simulink model "LUT_liver_pancreas_30"  (R2023b)
settings: Solver=FixedStepAuto  StartTime=0  StopTime=10.1  FixedStep=Timegap  RelTol=1e-3
model workspace (MAT data in the model file):
  T1_input = 1.34
(part 2 of 3)

== system LUT_liver_pancreas_30/If Action Subsystem6/If Action Subsystem1/If Action Subsystem6/If Action Subsystem3 ==
  In1 : Inport
  Action Port : ActionPort  ActionPortLabel=elseif( u1 >= 1.025)
  LUT 1.03RR : Lookup_n-D  NumberOfTableDimensions=1  BreakpointsForDimension1=[465.6797;513.9306;612.0294;710.55;809.0188;907.4097;1005.737;1104.014;1202.255;1300.466;1398.654;1496.822;1594.973;1693.109;1791.227;1889.324;1987.387]  Table=[400;500;600;700;800;900;1000;1100;1200;1300;1400;1500;1600;1700;1800;1900;2000]  InternalRulePriority=Speed  RndMeth=Simplest
  Out1 : Outport
  wires:
  In1/1 -> LUT 1.03RR/1
  LUT 1.03RR/1 -> Out1/1

== system LUT_liver_pancreas_30/If Action Subsystem6/If Action Subsystem1/If Action Subsystem6/If Action Subsystem4 ==
  In1 : Inport
  Action Port : ActionPort  ActionPortLabel=elseif( u1 >= 1.035)
  LUT 1.04RR : Lookup_n-D  NumberOfTableDimensions=1  BreakpointsForDimension1=[465.4805;513.7116;611.7076;710.1164;808.4681;906.7384;1004.942;1103.096;1201.21;1299.295;1397.356;1495.397;1593.421;1691.429;1789.421;1887.393;1985.334]  Table=[400;500;600;700;800;900;1000;1100;1200;1300;1400;1500;1600;1700;1800;1900;2000]  InternalRulePriority=Speed  RndMeth=Simplest
  Out1 : Outport
  wires:
  In1/1 -> LUT 1.04RR/1
  LUT 1.04RR/1 -> Out1/1

== system LUT_liver_pancreas_30/If Action Subsystem6/If Action Subsystem1/If Action Subsystem6/If Action Subsystem5 ==
  In1 : Inport
  Action Port : ActionPort  ActionPortLabel=elseif( u1 >= 1.055)
  LUT 1.06RR : Lookup_n-D  NumberOfTableDimensions=1  BreakpointsForDimension1=[465.091;513.2858;611.0845;709.278;807.4037;905.441;1003.407;1101.319;1199.191;1297.031;1394.845;1492.639;1590.416;1688.177;1785.923;1883.65;1981.353]  Table=[400;500;600;700;800;900;1000;1100;1200;1300;1400;1500;1600;1700;1800;1900;2000]  InternalRulePriority=Speed  RndMeth=Simplest
  Out1 : Outport
  wires:
  In1/1 -> LUT 1.06RR/1
  LUT 1.06RR/1 -> Out1/1

== system LUT_liver_pancreas_30/If Action Subsystem6/If Action Subsystem1/If Action Subsystem6/If Action Subsystem6 ==
  In1 : Inport
  Action Port : ActionPort  ActionPortLabel=elseif( u1 >= 1.045)
  LUT 1.05RR : Lookup_n-D  NumberOfTableDimensions=1  BreakpointsForDimension1=[465.2843;513.4967;611.3927;709.6925;807.9298;906.0823;1004.166;1102.198;1200.189;1298.15;1396.087;1494.003;1591.902;1689.785;1787.653;1885.502;1983.323]  Table=[400;500;600;700;800;900;1000;1100;1200;1300;1400;1500;1600;1700;1800;1900;2000]  InternalRulePriority=Speed  RndMeth=Simplest
  Out1 : Outport
  wires:
  In1/1 -> LUT 1.05RR/1
  LUT 1.05RR/1 -> Out1/1

== system LUT_liver_pancreas_30/If Action Subsystem6/If Action Subsystem1/If Action Subsystem6/If Action Subsystem7 ==
  In1 : Inport
  Action Port : ActionPort  ActionPortLabel=elseif( u1 >= 1.065)
  LUT 1.07RR : Lookup_n-D  NumberOfTableDimensions=1  BreakpointsForDimension1=[464.9007;513.0789;610.783;708.8729;806.8895;904.8142;1002.665;1100.461;1198.214;1295.935;1393.631;1491.305;1588.962;1686.603;1784.229;1881.838;1979.424]  Table=[400;500;600;700;800;900;1000;1100;1200;1300;1400;1500;1600;1700;1800;1900;2000]  InternalRulePriority=Speed  RndMeth=Simplest
  Out1 : Outport
  wires:
  In1/1 -> LUT 1.07RR/1
  LUT 1.07RR/1 -> Out1/1

== system LUT_liver_pancreas_30/If Action Subsystem6/If Action Subsystem1/If Action Subsystem6/If Action Subsystem8 ==
  In1 : Inport
  Action Port : ActionPort  ActionPortLabel=elseif(u1 >= 1.075)
  LUT 1.08RR : Lookup_n-D  NumberOfTableDimensions=1  BreakpointsForDimension1=[464.7133;512.876;610.4881;708.4768;806.3869;904.2015;1001.94;1099.622;1197.26;1294.864;1392.443;1490;1587.539;1685.063;1782.571;1880.063;1977.535]  Table=[400;500;600;700;800;900;1000;1100;1200;1300;1400;1500;1600;1700;1800;1900;2000]  InternalRulePriority=Speed  RndMeth=Simplest
  Out1 : Outport
  wires:
  In1/1 -> LUT 1.08RR/1
  LUT 1.08RR/1 -> Out1/1

== system LUT_liver_pancreas_30/If Action Subsystem6/If Action Subsystem1/If Action Subsystem6/If Action Subsystem9 ==
  In1 : Inport
  Action Port : ActionPort  ActionPortLabel=if(u1 >= 1.085)
  LUT 1.09RR : Lookup_n-D  NumberOfTableDimensions=1  BreakpointsForDimension1=[412.0667;553.6807;651.0883;748.3345;845.4429;942.4605;1039.419;1136.338;1233.23;1330.102;1426.961;1523.81;1620.651;1717.486;1814.317;1911.142;2007.964]  Table=[464.5288;512.6769;610.1995;708.0897;805.8957;903.6027;1001.231;1098.801;1196.326;1293.817;1391.281;1488.723;1586.147;1683.555;1780.949;1878.326;1975.684]  InternalRulePriority=Speed  RndMeth=Simplest
  Out1 : Outport
  wires:
  In1/1 -> LUT 1.09RR/1
  LUT 1.09RR/1 -> Out1/1

== system LUT_liver_pancreas_30/If Action Subsystem6/If Action Subsystem1/If Action Subsystem7/If Action Subsystem1 ==
  In1 : Inport
  Action Port : ActionPort  ActionPortLabel=elseif( u1 >= 1.215)
  LUT 1.22RR : Lookup_n-D  NumberOfTableDimensions=1  BreakpointsForDimension1=[462.3821;510.4145;606.9721;703.7795;800.4299;896.9327;993.3239;1089.632;1185.879;1282.079;1378.243;1474.378;1570.491;1666.584;1762.661;1858.723;1954.773]  Table=[400;500;600;700;800;900;1000;1100;1200;1300;1400;1500;1600;1700;1800;1900;2000]  InternalRulePriority=Speed  RndMeth=Simplest
  Out1 : Outport
  wires:
  In1/1 -> LUT 1.22RR/1
  LUT 1.22RR/1 -> Out1/1

== system LUT_liver_pancreas_30/If Action Subsystem6/If Action Subsystem1/If Action Subsystem7/If Action Subsystem10 ==
  In1 : Inport
  Action Port : ActionPort  ActionPortLabel=elseif( u1 >= 1.205)
  LUT 1.21RR : Lookup_n-D  NumberOfTableDimensions=1  BreakpointsForDimension1=[462.5316;510.5687;607.1891;704.0681;800.7958;897.3798;993.8548;1090.249;1186.583;1282.871;1379.124;1475.349;1571.551;1667.734;1763.902;1860.055;1956.195]  Table=[400;500;600;700;800;900;1000;1100;1200;1300;1400;1500;1600;1700;1800;1900;2000]  InternalRulePriority=Speed  RndMeth=Simplest
  Out1 : Outport
  wires:
  In1/1 -> LUT 1.21RR/1
  LUT 1.21RR/1 -> Out1/1

== system LUT_liver_pancreas_30/If Action Subsystem6/If Action Subsystem1/If Action Subsystem7/If Action Subsystem2 ==
  In1 : Inport
  Action Port : ActionPort  ActionPortLabel=else
  LUT 1.20RR : Lookup_n-D  NumberOfTableDimensions=1  BreakpointsForDimension1=[462.6836;510.7261;607.4108;704.3632;801.17;897.8369;994.3974;1090.879;1187.302;1283.68;1380.023;1476.339;1572.633;1668.908;1765.168;1861.413;1957.645]  Table=[400;500;600;700;800;900;1000;1100;1200;1300;1400;1500;1600;1700;1800;1900;2000]  InternalRulePriority=Speed  RndMeth=Simplest
  Out1 : Outport
  wires:
  In1/1 -> LUT 1.20RR/1
  LUT 1.20RR/1 -> Out1/1

== system LUT_liver_pancreas_30/If Action Subsystem6/If Action Subsystem1/If Action Subsystem7/If Action Subsystem3 ==
  In1 : Inport
  Action Port : ActionPort  ActionPortLabel=elseif( u1 >= 1.225)
  LUT 1.23RR : Lookup_n-D  NumberOfTableDimensions=1  BreakpointsForDimension1=[462.235;510.2632;606.7599;703.4974;800.072;896.4954;992.8044;1089.029;1185.19;1281.304;1377.38;1473.428;1569.452;1665.456;1761.444;1857.418;1953.378]  Table=[400;500;600;700;800;900;1000;1100;1200;1300;1400;1500;1600;1700;1800;1900;2000]  InternalRulePriority=Speed  RndMeth=Simplest
  Out1 : Outport
  wires:
  In1/1 -> LUT 1.23RR/1
  LUT 1.23RR/1 -> Out1/1

== system LUT_liver_pancreas_30/If Action Subsystem6/If Action Subsystem1/If Action Subsystem7/If Action Subsystem4 ==
  In1 : Inport
  Action Port : ActionPort  ActionPortLabel=elseif( u1 >= 1.235)
  LUT 1.24RR : Lookup_n-D  NumberOfTableDimensions=1  BreakpointsForDimension1=[462.0903;510.1148;606.5523;703.2214;799.7221;896.0676;992.296;1088.438;1184.516;1280.544;1376.535;1472.496;1568.433;1664.351;1760.251;1856.137;1952.01]  Table=[400;500;600;700;800;900;1000;1100;1200;1300;1400;1500;1600;1700;1800;1900;2000]  InternalRulePriority=Speed  RndMeth=Simplest
  Out1 : Outport
  wires:
  In1/1 -> LUT 1.24RR/1
  LUT 1.24RR/1 -> Out1/1

== system LUT_liver_pancreas_30/If Action Subsystem6/If Action Subsystem1/If Action Subsystem7/If Action Subsystem5 ==
  In1 : Inport
  Action Port : ActionPort  ActionPortLabel=elseif( u1 >= 1.255)
  LUT 1.26RR : Lookup_n-D  NumberOfTableDimensions=1  BreakpointsForDimension1=[461.8078;509.8267;606.1502;702.6876;799.045;895.2396;991.3117;1087.293;1183.208;1279.071;1374.896;1470.689;1566.457;1662.204;1757.935;1853.651;1949.353]  Table=[400;500;600;700;800;900;1000;1100;1200;1300;1400;1500;1600;1700;1800;1900;2000]  InternalRulePriority=Speed  RndMeth=Simplest
  Out1 : Outport
  wires:
  In1/1 -> LUT 1.26RR/1
  LUT 1.26RR/1 -> Out1/1

== system LUT_liver_pancreas_30/If Action Subsystem6/If Action Subsystem1/If Action Subsystem7/If Action Subsystem6 ==
  In1 : Inport
  Action Port : ActionPort  ActionPortLabel=elseif( u1 >= 1.245)
  LUT 1.25RR : Lookup_n-D  NumberOfTableDimensions=1  BreakpointsForDimension1=[461.9479;509.9694;606.349;702.9515;799.3798;895.6491;991.7985;1087.86;1183.855;1279.8;1375.707;1471.583;1567.435;1663.267;1759.082;1854.882;1950.669]  Table=[400;500;600;700;800;900;1000;1100;1200;1300;1400;1500;1600;1700;1800;1900;2000]  InternalRulePriority=Speed  RndMeth=Simplest
  Out1 : Outport
  wires:
  In1/1 -> LUT 1.25RR/1
  LUT 1.25RR/1 -> Out1/1

== system LUT_liver_pancreas_30/If Action Subsystem6/If Action Subsystem1/If Action Subsystem7/If Action Subsystem7 ==
  In1 : Inport
  Action Port : ActionPort  ActionPortLabel=elseif( u1 >= 1.265)
  LUT 1.27RR : Lookup_n-D  NumberOfTableDimensions=1  BreakpointsForDimension1=[461.6699;509.6867;605.9556;702.4294;798.7176;894.839;990.8352;1086.739;1182.574;1278.357;1374.1;1469.812;1565.498;1661.163;1756.81;1852.443;1948.062]  Table=[400;500;600;700;800;900;1000;1100;1200;1300;1400;1500;1600;1700;1800;1900;2000]  InternalRulePriority=Speed  RndMeth=Simplest
  Out1 : Outport
  wires:
  In1/1 -> LUT 1.27RR/1
  LUT 1.27RR/1 -> Out1/1

== system LUT_liver_pancreas_30/If Action Subsystem6/If Action Subsystem1/If Action Subsystem7/If Action Subsystem8 ==
  In1 : Inport
  Action Port : ActionPort  ActionPortLabel=elseif(u1 >= 1.275)
  LUT 1.28RR : Lookup_n-D  NumberOfTableDimensions=1  BreakpointsForDimension1=[461.5343;509.5495;605.7652;702.1769;798.3973;894.447;990.3687;1086.196;1181.954;1277.658;1373.321;1468.952;1564.557;1660.141;1755.707;1851.258;1946.796]  Table=[400;500;600;700;800;900;1000;1100;1200;1300;1400;1500;1600;1700;1800;1900;2000]  InternalRulePriority=Speed  RndMeth=Simplest
  Out1 : Outport
  wires:
  In1/1 -> LUT 1.28RR/1
  LUT 1.28RR/1 -> Out1/1

== system LUT_liver_pancreas_30/If Action Subsystem6/If Action Subsystem1/If Action Subsystem7/If Action Subsystem9 ==
  In1 : Inport
  Action Port : ActionPort  ActionPortLabel=if(u1 >= 1.285)
  LUT 1.29RR : Lookup_n-D  NumberOfTableDimensions=1  BreakpointsForDimension1=[461.4008;509.4148;605.5788;701.9299;798.084;894.0634;989.9122;1085.665;1181.346;1276.973;1372.558;1468.11;1563.635;1659.139;1754.625;1850.096;1945.553]  Table=[400;500;600;700;800;900;1000;1100;1200;1300;1400;1500;1600;1700;1800;1900;2000]  InternalRulePriority=Speed  RndMeth=Simplest
  Out1 : Outport
  wires:
  In1/1 -> LUT 1.29RR/1
  LUT 1.29RR/1 -> Out1/1

== system LUT_liver_pancreas_30/If Action Subsystem6/If Action Subsystem1/If Action Subsystem8/If Action Subsystem1 ==
  In1 : Inport
  Action Port : ActionPort  ActionPortLabel=elseif( u1 >= 1.315)
  LUT 1.32RR : Lookup_n-D  NumberOfTableDimensions=1  BreakpointsForDimension1=[461.0128;509.0261;605.043;701.2207;797.1841;892.9612;988.5993;1084.135;1179.595;1274.998;1370.356;1465.679;1560.975;1656.247;1751.501;1846.739;1941.963]  Table=[400;500;600;700;800;900;1000;1100;1200;1300;1400;1500;1600;1700;1800;1900;2000]  InternalRulePriority=Speed  RndMeth=Simplest
  Out1 : Outport
  wires:
  In1/1 -> LUT 1.32RR/1
  LUT 1.32RR/1 -> Out1/1

== system LUT_liver_pancreas_30/If Action Subsystem6/If Action Subsystem1/If Action Subsystem8/If Action Subsystem10 ==
  In1 : Inport
  Action Port : ActionPort  ActionPortLabel=elseif( u1 >= 1.305)
  LUT 1.31RR : Lookup_n-D  NumberOfTableDimensions=1  BreakpointsForDimension1=[461.1401;509.1532;605.2178;701.452;797.4775;893.3207;989.0277;1084.635;1180.167;1275.643;1371.075;1466.474;1561.844;1657.193;1752.523;1847.837;1943.137]  Table=[400;500;600;700;800;900;1000;1100;1200;1300;1400;1500;1600;1700;1800;1900;2000]  InternalRulePriority=Speed  RndMeth=Simplest
  Out1 : Outport
  wires:
  In1/1 -> LUT 1.31RR/1
  LUT 1.31RR/1 -> Out1/1

== system LUT_liver_pancreas_30/If Action Subsystem6/If Action Subsystem1/If Action Subsystem8/If Action Subsystem2 ==
  In1 : Inport
  Action Port : ActionPort  ActionPortLabel=else
  LUT 1.30RR : Lookup_n-D  NumberOfTableDimensions=1  BreakpointsForDimension1=[461.2694;509.2828;605.3963;701.6863;797.7774;893.688;989.4652;1085.144;1180.75;1276.301;1371.809;1467.283;1562.731;1658.157;1753.564;1848.956;1944.334]  Table=[400;500;600;700;800;900;1000;1100;1200;1300;1400;1500;1600;1700;1800;1900;2000]  InternalRulePriority=Speed  RndMeth=Simplest
  Out1 : Outport
  wires:
  In1/1 -> LUT 1.30RR/1
  LUT 1.30RR/1 -> Out1/1

== system LUT_liver_pancreas_30/If Action Subsystem6/If Action Subsystem1/If Action Subsystem8/If Action Subsystem3 ==
  In1 : Inport
  Action Port : ActionPort  ActionPortLabel=elseif( u1 >= 1.325)
  LUT 1.33RR : Lookup_n-D  NumberOfTableDimensions=1  BreakpointsForDimension1=[460.8876;508.9014;604.8719;700.9945;796.897;892.6093;988.1798;1083.646;1179.035;1274.366;1369.651;1464.9;1560.122;1655.32;1750.499;1845.662;1940.81]  Table=[400;500;600;700;800;900;1000;1100;1200;1300;1400;1500;1600;1700;1800;1900;2000]  InternalRulePriority=Speed  RndMeth=Simplest
  Out1 : Outport
  wires:
  In1/1 -> LUT 1.33RR/1
  LUT 1.33RR/1 -> Out1/1

== system LUT_liver_pancreas_30/If Action Subsystem6/If Action Subsystem1/If Action Subsystem8/If Action Subsystem4 ==
  In1 : Inport
  Action Port : ActionPort  ActionPortLabel=elseif( u1 >= 1.335)
  LUT 1.34RR : Lookup_n-D  NumberOfTableDimensions=1  BreakpointsForDimension1=[460.7643;508.779;604.7044;700.7732;796.6161;892.2649;987.7691;1083.167;1178.486;1273.746;1368.959;1464.137;1559.285;1654.41;1749.515;1844.604;1939.678]  Table=[400;500;600;700;800;900;1000;1100;1200;1300;1400;1500;1600;1700;1800;1900;2000]  InternalRulePriority=Speed  RndMeth=Simplest
  Out1 : Outport
  wires:
  In1/1 -> LUT 1.34RR/1
  LUT 1.34RR/1 -> Out1/1

== system LUT_liver_pancreas_30/If Action Subsystem6/If Action Subsystem1/If Action Subsystem8/If Action Subsystem5 ==
  In1 : Inport
  Action Port : ActionPort  ActionPortLabel=elseif( u1 >= 1.355)
  LUT 1.36RR : Lookup_n-D  NumberOfTableDimensions=1  BreakpointsForDimension1=[460.5234;508.5411;604.3798;700.3447;796.0723;891.5977;986.9731;1082.238;1177.422;1272.543;1367.616;1462.652;1557.658;1652.64;1747.602;1842.547;1937.477]  Table=[400;500;600;700;800;900;1000;1100;1200;1300;1400;1500;1600;1700;1800;1900;2000]  InternalRulePriority=Speed  RndMeth=Simplest
  Out1 : Outport
  wires:
  In1/1 -> LUT 1.36RR/1
  LUT 1.36RR/1 -> Out1/1

== system LUT_liver_pancreas_30/If Action Subsystem6/If Action Subsystem1/If Action Subsystem8/If Action Subsystem6 ==
  In1 : Inport
  Action Port : ActionPort  ActionPortLabel=elseif( u1 >= 1.345)
  LUT 1.35RR : Lookup_n-D  NumberOfTableDimensions=1  BreakpointsForDimension1=[460.6429;508.6589;604.5404;700.5566;796.3413;891.9277;987.3669;1082.698;1177.949;1273.138;1368.281;1463.387;1558.464;1653.517;1748.55;1843.566;1938.567]  Table=[400;500;600;700;800;900;1000;1100;1200;1300;1400;1500;1600;1700;1800;1900;2000]  InternalRulePriority=Speed  RndMeth=Simplest
  Out1 : Outport
  wires:
  In1/1 -> LUT 1.35RR/1
  LUT 1.35RR/1 -> Out1/1

== system LUT_liver_pancreas_30/If Action Subsystem6/If Action Subsystem1/If Action Subsystem8/If Action Subsystem7 ==
  In1 : Inport
  Action Port : ActionPort  ActionPortLabel=elseif( u1 >= 1.365)
  LUT 1.37RR : Lookup_n-D  NumberOfTableDimensions=1  BreakpointsForDimension1=[460.4057;508.4254;604.2226;700.1373;795.809;891.2746;986.5873;1081.788;1176.905;1271.959;1366.964;1461.932;1556.868;1651.78;1746.672;1841.546;1936.405]  Table=[400;500;600;700;800;900;1000;1100;1200;1300;1400;1500;1600;1700;1800;1900;2000]  InternalRulePriority=Speed  RndMeth=Simplest
  Out1 : Outport
  wires:
  In1/1 -> LUT 1.37RR/1
  LUT 1.37RR/1 -> Out1/1

== system LUT_liver_pancreas_30/If Action Subsystem6/If Action Subsystem1/If Action Subsystem8/If Action Subsystem8 ==
  In1 : Inport
  Action Port : ActionPort  ActionPortLabel=elseif(u1 >= 1.375)
  LUT 1.38RR : Lookup_n-D  NumberOfTableDimensions=1  BreakpointsForDimension1=[460.2899;508.3119;604.0687;699.9344;795.5514;890.9583;986.2096;1081.347;1176.399;1271.386;1366.325;1461.224;1556.093;1650.936;1745.758;1840.564;1935.354]  Table=[400;500;600;700;800;900;1000;1100;1200;1300;1400;1500;1600;1700;1800;1900;2000]  InternalRulePriority=Speed  RndMeth=Simplest
  Out1 : Outport
  wires:
  In1/1 -> LUT 1.38RR/1
  LUT 1.38RR/1 -> Out1/1

== system LUT_liver_pancreas_30/If Action Subsystem6/If Action Subsystem1/If Action Subsystem8/If Action Subsystem9 ==
  In1 : Inport
  Action Port : ActionPort  ActionPortLabel=if(u1 >= 1.385)
  LUT 1.39RR : Lookup_n-D  NumberOfTableDimensions=1  BreakpointsForDimension1=[460.1758;508.2005;603.9179;699.7359;795.2993;890.6487;985.8396;1080.914;1175.902;1270.825;1365.698;1460.53;1555.332;1650.107;1744.862;1839.599;1934.321]  Table=[400;500;600;700;800;900;1000;1100;1200;1300;1400;1500;1600;1700;1800;1900;2000]  InternalRulePriority=Speed  RndMeth=Simplest
  Out1 : Outport
  wires:
  In1/1 -> LUT 1.39RR/1
  LUT 1.39RR/1 -> Out1/1

== system LUT_liver_pancreas_30/If Action Subsystem6/If Action Subsystem1/If Action Subsystem9/If Action Subsystem1 ==
  In1 : Inport
  Action Port : ActionPort  ActionPortLabel=elseif( u1 >= 1.415)
  LUT 1.42RR : Lookup_n-D  NumberOfTableDimensions=1  BreakpointsForDimension1=[459.8439;507.8784;603.4841;699.1652;794.5746;889.758;984.7744;1079.668;1174.471;1269.205;1363.886;1458.526;1553.132;1647.711;1742.269;1836.807;1931.33]  Table=[400;500;600;700;800;900;1000;1100;1200;1300;1400;1500;1600;1700;1800;1900;2000]  InternalRulePriority=Speed  RndMeth=Simplest
  Out1 : Outport
  wires:
  In1/1 -> LUT 1.42RR/1
  LUT 1.42RR/1 -> Out1/1

== system LUT_liver_pancreas_30/If Action Subsystem6/If Action Subsystem1/If Action Subsystem9/If Action Subsystem10 ==
  In1 : Inport
  Action Port : ActionPort  ActionPortLabel=elseif( u1 >= 1.405)
  LUT 1.41RR : Lookup_n-D  NumberOfTableDimensions=1  BreakpointsForDimension1=[459.9529;507.9838;603.6257;699.3513;794.811;890.0486;985.1221;1080.075;1174.939;1269.735;1364.479;1459.181;1553.852;1648.495;1743.117;1837.721;1932.309]  Table=[400;500;600;700;800;900;1000;1100;1200;1300;1400;1500;1600;1700;1800;1900;2000]  InternalRulePriority=Speed  RndMeth=Simplest
  Out1 : Outport
  wires:
  In1/1 -> LUT 1.41RR/1
  LUT 1.41RR/1 -> Out1/1

== system LUT_liver_pancreas_30/If Action Subsystem6/If Action Subsystem1/If Action Subsystem9/If Action Subsystem2 ==
  In1 : Inport
  Action Port : ActionPort  ActionPortLabel=else
  LUT 1.40RR : Lookup_n-D  NumberOfTableDimensions=1  BreakpointsForDimension1=[460.0635;508.0912;603.7703;699.5415;795.0525;890.3455;985.4771;1080.49;1175.416;1270.275;1365.082;1459.85;1554.585;1649.294;1743.982;1838.651;1933.306]  Table=[400;500;600;700;800;900;1000;1100;1200;1300;1400;1500;1600;1700;1800;1900;2000]  InternalRulePriority=Speed  RndMeth=Simplest
  Out1 : Outport
  wires:
  In1/1 -> LUT 1.40RR/1
  LUT 1.40RR/1 -> Out1/1

== system LUT_liver_pancreas_30/If Action Subsystem6/If Action Subsystem1/If Action Subsystem9/If Action Subsystem3 ==
  In1 : Inport
  Action Port : ActionPort  ActionPortLabel=elseif( u1 >= 1.425)
  LUT 1.43RR : Lookup_n-D  NumberOfTableDimensions=1  BreakpointsForDimension1=[459.7366;507.7749;603.3454;698.9829;794.3431;889.4733;984.4337;1079.27;1174.013;1268.686;1363.305;1457.882;1552.426;1646.942;1741.435;1835.91;1930.368]  Table=[400;500;600;700;800;900;1000;1100;1200;1300;1400;1500;1600;1700;1800;1900;2000]  InternalRulePriority=Speed  RndMeth=Simplest
  Out1 : Outport
  wires:
  In1/1 -> LUT 1.43RR/1
  LUT 1.43RR/1 -> Out1/1

== system LUT_liver_pancreas_30/If Action Subsystem6/If Action Subsystem1/If Action Subsystem9/If Action Subsystem4 ==
  In1 : Inport
  Action Port : ActionPort  ActionPortLabel=elseif( u1 >= 1.435)
  LUT 1.44RR : Lookup_n-D  NumberOfTableDimensions=1  BreakpointsForDimension1=[459.6309;507.6733;603.2096;698.8046;794.1166;889.1946;984.1;1078.879;1173.563;1268.177;1362.735;1457.251;1551.732;1646.186;1740.616;1835.028;1929.423]  Table=[400;500;600;700;800;900;1000;1100;1200;1300;1400;1500;1600;1700;1800;1900;2000]  InternalRulePriority=Speed  RndMeth=Simplest
  Out1 : Outport
  wires:
  In1/1 -> LUT 1.44RR/1
  LUT 1.44RR/1 -> Out1/1

== system LUT_liver_pancreas_30/If Action Subsystem6/If Action Subsystem1/If Action Subsystem9/If Action Subsystem5 ==
  In1 : Inport
  Action Port : ActionPort  ActionPortLabel=elseif( u1 >= 1.455)
  LUT 1.46RR : Lookup_n-D  NumberOfTableDimensions=1  BreakpointsForDimension1=[459.4241;507.4755;602.9462;698.4591;793.6778;888.6544;983.4526;1078.12;1172.69;1267.187;1361.627;1456.023;1550.383;1644.714;1739.022;1833.311;1927.583]  Table=[400;500;600;700;800;900;1000;1100;1200;1300;1400;1500;1600;1700;1800;1900;2000]  InternalRulePriority=Speed  RndMeth=Simplest
  Out1 : Outport
  wires:
  In1/1 -> LUT 1.46RR/1
  LUT 1.46RR/1 -> Out1/1

== system LUT_liver_pancreas_30/If Action Subsystem6/If Action Subsystem1/If Action Subsystem9/If Action Subsystem6 ==
  In1 : Inport
  Action Port : ActionPort  ActionPortLabel=elseif( u1 >= 1.445)
  LUT 1.45RR : Lookup_n-D  NumberOfTableDimensions=1  BreakpointsForDimension1=[459.5267;507.5735;603.0765;698.63;793.8948;888.9217;983.773;1078.496;1173.123;1267.677;1362.176;1456.631;1551.051;1645.443;1739.812;1834.162;1928.495]  Table=[400;500;600;700;800;900;1000;1100;1200;1300;1400;1500;1600;1700;1800;1900;2000]  InternalRulePriority=Speed  RndMeth=Simplest
  Out1 : Outport
  wires:
  In1/1 -> LUT 1.45RR/1
  LUT 1.45RR/1 -> Out1/1

== system LUT_liver_pancreas_30/If Action Subsystem6/If Action Subsystem1/If Action Subsystem9/If Action Subsystem7 ==
  In1 : Inport
  Action Port : ActionPort  ActionPortLabel=elseif( u1 >= 1.465)
  LUT 1.47RR : Lookup_n-D  NumberOfTableDimensions=1  BreakpointsForDimension1=[459.323;507.3793;602.8185;698.2919;793.4652;888.3926;983.1387;1077.752;1172.266;1266.706;1361.088;1455.425;1549.727;1643.999;1738.247;1832.475;1926.686]  Table=[400;500;600;700;800;900;1000;1100;1200;1300;1400;1500;1600;1700;1800;1900;2000]  InternalRulePriority=Speed  RndMeth=Simplest
  Out1 : Outport
  wires:
  In1/1 -> LUT 1.47RR/1
  LUT 1.47RR/1 -> Out1/1

== system LUT_liver_pancreas_30/If Action Subsystem6/If Action Subsystem1/If Action Subsystem9/If Action Subsystem8 ==
  In1 : Inport
  Action Port : ActionPort  ActionPortLabel=elseif(u1 >= 1.475)
  LUT 1.48RR : Lookup_n-D  NumberOfTableDimensions=1  BreakpointsForDimension1=[459.2234;507.2847;602.6934;698.1281;793.2572;888.1363;982.8312;1077.391;1171.851;1266.235;1360.56;1454.839;1549.082;1643.295;1737.484;1831.653;1925.805]  Table=[400;500;600;700;800;900;1000;1100;1200;1300;1400;1500;1600;1700;1800;1900;2000]  InternalRulePriority=Speed  RndMeth=Simplest
  Out1 : Outport
  wires:
  In1/1 -> LUT 1.48RR/1
  LUT 1.48RR/1 -> Out1/1

== system LUT_liver_pancreas_30/If Action Subsystem6/If Action Subsystem1/If Action Subsystem9/If Action Subsystem9 ==
  In1 : Inport
  Action Port : ActionPort  ActionPortLabel=if(u1 >= 1.485)
  LUT 1.49RR : Lookup_n-D  NumberOfTableDimensions=1  BreakpointsForDimension1=[459.1252;507.1919;602.5709;697.9678;793.0535;887.8852;982.5299;1077.037;1171.443;1265.772;1360.041;1454.264;1548.449;1642.605;1736.735;1830.846;1924.939]  Table=[400;500;600;700;800;900;1000;1100;1200;1300;1400;1500;1600;1700;1800;1900;2000]  InternalRulePriority=Speed  RndMeth=Simplest
  Out1 : Outport
  wires:
  In1/1 -> LUT 1.49RR/1
  LUT 1.49RR/1 -> Out1/1

== system LUT_liver_pancreas_30/If Action Subsystem6/If Action Subsystem2/If Action Subsystem5/If Action Subsystem1 ==
  In1 : Inport
  Action Port : ActionPort  ActionPortLabel=elseif( u1 >= 1.615)
  LUT 1.62RR : Lookup_n-D  NumberOfTableDimensions=1  BreakpointsForDimension1=[457.9682;506.1215;601.1841;696.1646;790.7619;885.0533;979.1199;1073.022;1166.801;1260.486;1354.101;1447.659;1541.172;1634.649;1728.096;1821.519;1914.921]  Table=[400;500;600;700;800;900;1000;1100;1200;1300;1400;1500;1600;1700;1800;1900;2000]  InternalRulePriority=Speed  RndMeth=Simplest
  Out1 : Outport
  wires:
  In1/1 -> LUT 1.62RR/1
  LUT 1.62RR/1 -> Out1/1

== system LUT_liver_pancreas_30/If Action Subsystem6/If Action Subsystem2/If Action Subsystem5/If Action Subsystem10 ==
  In1 : Inport
  Action Port : ActionPort  ActionPortLabel=elseif( u1>= 1.605)
  LUT 1.61RR : Lookup_n-D  NumberOfTableDimensions=1  BreakpointsForDimension1=[458.05;506.1956;601.2784;696.2865;790.9167;885.2451;979.3517;1073.295;1167.118;1260.849;1354.509;1448.114;1541.674;1635.199;1728.694;1822.165;1915.616]  Table=[400;500;600;700;800;900;1000;1100;1200;1300;1400;1500;1600;1700;1800;1900;2000]  InternalRulePriority=Speed  RndMeth=Simplest
  Out1 : Outport
  wires:
  In1/1 -> LUT 1.61RR/1
  LUT 1.61RR/1 -> Out1/1

== system LUT_liver_pancreas_30/If Action Subsystem6/If Action Subsystem2/If Action Subsystem5/If Action Subsystem2 ==
  In1 : Inport
  Action Port : ActionPort  ActionPortLabel=else
  LUT 1.60RR : Lookup_n-D  NumberOfTableDimensions=1  BreakpointsForDimension1=[458.1329;506.271;601.3746;696.4109;791.0749;885.441;979.5882;1073.575;1167.442;1261.218;1354.925;1448.577;1542.185;1635.759;1729.303;1822.823;1916.324]  Table=[400;500;600;700;800;900;1000;1100;1200;1300;1400;1500;1600;1700;1800;1900;2000]  InternalRulePriority=Speed  RndMeth=Simplest
  Out1 : Outport
  wires:
  In1/1 -> LUT 1.60RR/1
  LUT 1.60RR/1 -> Out1/1

== system LUT_liver_pancreas_30/If Action Subsystem6/If Action Subsystem2/If Action Subsystem5/If Action Subsystem3 ==
  In1 : Inport
  Action Port : ActionPort  ActionPortLabel=elseif( u1 >= 1.625)
  LUT 1.63RR : Lookup_n-D  NumberOfTableDimensions=1  BreakpointsForDimension1=[457.8875;506.0486;601.0917;696.0453;790.6102;884.8653;978.8927;1072.753;1166.489;1260.131;1353.7;1447.211;1540.678;1634.108;1727.507;1820.882;1914.236]  Table=[400;500;600;700;800;900;1000;1100;1200;1300;1400;1500;1600;1700;1800;1900;2000]  InternalRulePriority=Speed  RndMeth=Simplest
  Out1 : Outport
  wires:
  In1/1 -> LUT 1.63RR/1
  LUT 1.63RR/1 -> Out1/1

== system LUT_liver_pancreas_30/If Action Subsystem6/If Action Subsystem2/If Action Subsystem5/If Action Subsystem4 ==
  In1 : Inport
  Action Port : ActionPort  ActionPortLabel=elseif( u1 >= 1.635)
  LUT 1.64RR : Lookup_n-D  NumberOfTableDimensions=1  BreakpointsForDimension1=[457.8079;505.9769;601.001;695.9284;790.4617;884.6812;978.6701;1072.49;1166.183;1259.781;1353.306;1446.772;1540.193;1633.576;1726.929;1820.257;1913.563]  Table=[400;500;600;700;800;900;1000;1100;1200;1300;1400;1500;1600;1700;1800;1900;2000]  InternalRulePriority=Speed  RndMeth=Simplest
  Out1 : Outport
  wires:
  In1/1 -> LUT 1.64RR/1
  LUT 1.64RR/1 -> Out1/1

== system LUT_liver_pancreas_30/If Action Subsystem6/If Action Subsystem2/If Action Subsystem5/If Action Subsystem5 ==
  In1 : Inport
  Action Port : ActionPort  ActionPortLabel=elseif( u1 >= 1.655)
  LUT 1.66RR : Lookup_n-D  NumberOfTableDimensions=1  BreakpointsForDimension1=[457.6519;505.837;600.8251;695.7019;790.1739;884.3242;978.238;1071.978;1165.589;1259.102;1352.539;1445.917;1539.247;1632.539;1725.8;1819.036;1912.249]  Table=[400;500;600;700;800;900;1000;1100;1200;1300;1400;1500;1600;1700;1800;1900;2000]  InternalRulePriority=Speed  RndMeth=Simplest
  Out1 : Outport
  wires:
  In1/1 -> LUT 1.66RR/1
  LUT 1.66RR/1 -> Out1/1

== system LUT_liver_pancreas_30/If Action Subsystem6/If Action Subsystem2/If Action Subsystem5/If Action Subsystem6 ==
  In1 : Inport
  Action Port : ActionPort  ActionPortLabel=elseif( u1 >= 1.645)
  LUT 1.65RR : Lookup_n-D  NumberOfTableDimensions=1  BreakpointsForDimension1=[457.7294;505.9064;600.9122;695.8139;790.3163;884.5009;978.4519;1072.231;1165.883;1259.438;1352.919;1446.341;1539.716;1633.053;1726.36;1819.641;1912.901]  Table=[400;500;600;700;800;900;1000;1100;1200;1300;1400;1500;1600;1700;1800;1900;2000]  InternalRulePriority=Speed  RndMeth=Simplest
  Out1 : Outport
  wires:
  In1/1 -> LUT 1.65RR/1
  LUT 1.65RR/1 -> Out1/1

== system LUT_liver_pancreas_30/If Action Subsystem6/If Action Subsystem2/If Action Subsystem5/If Action Subsystem7 ==
  In1 : Inport
  Action Port : ActionPort  ActionPortLabel=elseif( u1 >= 1.665)
  LUT 1.67RR : Lookup_n-D  NumberOfTableDimensions=1  BreakpointsForDimension1=[457.5754;505.7688;600.7396;695.5921;790.0345;884.1511;978.0284;1071.73;1165.3;1258.771;1352.166;1445.5;1538.786;1632.034;1725.25;1818.44;1911.608]  Table=[400;500;600;700;800;900;1000;1100;1200;1300;1400;1500;1600;1700;1800;1900;2000]  InternalRulePriority=Speed  RndMeth=Simplest
  Out1 : Outport
  wires:
  In1/1 -> LUT 1.67RR/1
  LUT 1.67RR/1 -> Out1/1

== system LUT_liver_pancreas_30/If Action Subsystem6/If Action Subsystem2/If Action Subsystem5/If Action Subsystem8 ==
  In1 : Inport
  Action Port : ActionPort  ActionPortLabel=elseif(u1 >= 1.675)
  LUT 1.68RR : Lookup_n-D  NumberOfTableDimensions=1  BreakpointsForDimension1=[457.4999;505.7017;600.6559;695.4847;789.898;883.9816;977.8229;1071.486;1165.017;1258.447;1351.799;1445.091;1538.334;1631.537;1724.709;1817.854;1910.977]  Table=[400;500;600;700;800;900;1000;1100;1200;1300;1400;1500;1600;1700;1800;1900;2000]  InternalRulePriority=Speed  RndMeth=Simplest
  Out1 : Outport
  wires:
  In1/1 -> LUT 1.68RR/1
  LUT 1.68RR/1 -> Out1/1

== system LUT_liver_pancreas_30/If Action Subsystem6/If Action Subsystem2/If Action Subsystem5/If Action Subsystem9 ==
  In1 : Inport
  Action Port : ActionPort  ActionPortLabel=if(u1 >= 1.685)
  LUT 1.69RR : Lookup_n-D  NumberOfTableDimensions=1  BreakpointsForDimension1=[457.4253;505.6357;600.5738;695.3794;789.7643;883.8156;977.6216;1071.247;1164.739;1258.128;1351.439;1444.689;1537.889;1631.049;1724.177;1817.278;1910.357]  Table=[400;500;600;700;800;900;1000;1100;1200;1300;1400;1500;1600;1700;1800;1900;2000]  InternalRulePriority=Speed  RndMeth=Simplest
  Out1 : Outport
  wires:
  In1/1 -> LUT 1.69RR/1
  LUT 1.69RR/1 -> Out1/1

== system LUT_liver_pancreas_30/If Action Subsystem6/If Action Subsystem2/If Action Subsystem6/If Action Subsystem1 ==
  In1 : Inport
  Action Port : ActionPort  ActionPortLabel=elseif( u1 >= 1.515)
  LUT 1.52RR : Lookup_n-D  NumberOfTableDimensions=1  BreakpointsForDimension1=[458.839;506.923;602.2178;697.5067;792.4676;887.1625;981.6617;1076.017;1170.267;1264.435;1358.541;1452.599;1546.617;1640.604;1734.566;1828.506;1922.428]  Table=[400;500;600;700;800;900;1000;1100;1200;1300;1400;1500;1600;1700;1800;1900;2000]  InternalRulePriority=Speed  RndMeth=Simplest
  Out1 : Outport
  wires:
  In1/1 -> LUT 1.52RR/1
  LUT 1.52RR/1 -> Out1/1

== system LUT_liver_pancreas_30/If Action Subsystem6/If Action Subsystem2/If Action Subsystem6/If Action Subsystem10 ==
  In1 : Inport
  Action Port : ActionPort  ActionPortLabel=elseif( u1 >= 1.505)
  LUT 1.51RR : Lookup_n-D  NumberOfTableDimensions=1  BreakpointsForDimension1=[458.933;507.011;602.3331;697.6572;792.6588;887.3984;981.9452;1076.351;1170.651;1264.872;1359.032;1453.144;1547.217;1641.259;1735.276;1829.272;1923.251]  Table=[400;500;600;700;800;900;1000;1100;1200;1300;1400;1500;1600;1700;1800;1900;2000]  InternalRulePriority=Speed  RndMeth=Simplest
  Out1 : Outport
  wires:
  In1/1 -> LUT 1.51RR/1
  LUT 1.51RR/1 -> Out1/1

== system LUT_liver_pancreas_30/If Action Subsystem6/If Action Subsystem2/If Action Subsystem6/If Action Subsystem2 ==
  In1 : Inport
  Action Port : ActionPort  ActionPortLabel=else
  LUT 1.50RR : Lookup_n-D  NumberOfTableDimensions=1  BreakpointsForDimension1=[459.0284;507.1006;602.4508;697.8108;792.854;887.6393;982.2346;1076.691;1171.043;1265.318;1359.532;1453.698;1547.827;1641.926;1736;1830.052;1924.087]  Table=[400;500;600;700;800;900;1000;1100;1200;1300;1400;1500;1600;1700;1800;1900;2000]  InternalRulePriority=Speed  RndMeth=Simplest
  Out1 : Outport
  wires:
  In1/1 -> LUT 1.50RR/1
  LUT 1.50RR/1 -> Out1/1

== system LUT_liver_pancreas_30/If Action Subsystem6/If Action Subsystem2/If Action Subsystem6/If Action Subsystem3 ==
  In1 : Inport
  Action Port : ActionPort  ActionPortLabel=elseif( u1 >= 1.525)
  LUT 1.53RR : Lookup_n-D  NumberOfTableDimensions=1  BreakpointsForDimension1=[458.7464;506.8364;602.1048;697.3594;792.2804;886.9314;981.3838;1075.691;1169.889;1264.006;1358.06;1452.064;1546.028;1639.961;1733.868;1827.753;1921.619]  Table=[400;500;600;700;800;900;1000;1100;1200;1300;1400;1500;1600;1700;1800;1900;2000]  InternalRulePriority=Speed  RndMeth=Simplest
  Out1 : Outport
  wires:
  In1/1 -> LUT 1.53RR/1
  LUT 1.53RR/1 -> Out1/1

== system LUT_liver_pancreas_30/If Action Subsystem6/If Action Subsystem2/If Action Subsystem6/If Action Subsystem4 ==
  In1 : Inport
  Action Port : ActionPort  ActionPortLabel=elseif( u1 >= 1.535)
  LUT 1.54RR : Lookup_n-D  NumberOfTableDimensions=1  BreakpointsForDimension1=[458.655;506.7514;601.9941;697.2152;792.0971;886.7051;981.1115;1075.37;1169.519;1263.585;1357.587;1451.538;1545.45;1639.329;1733.181;1827.012;1920.824]  Table=[400;500;600;700;800;900;1000;1100;1200;1300;1400;1500;1600;1700;1800;1900;2000]  InternalRulePriority=Speed  RndMeth=Simplest
  Out1 : Outport
  wires:
  In1/1 -> LUT 1.54RR/1
  LUT 1.54RR/1 -> Out1/1

== system LUT_liver_pancreas_30/If Action Subsystem6/If Action Subsystem2/If Action Subsystem6/If Action Subsystem5 ==
  In1 : Inport
  Action Port : ActionPort  ActionPortLabel=elseif( u1 >= 1.555)
  LUT 1.56RR : Lookup_n-D  NumberOfTableDimensions=1  BreakpointsForDimension1=[458.4761;506.5857;601.7793;696.9358;791.7419;886.2662;980.5831;1074.748;1168.8;1262.766;1356.667;1450.515;1544.323;1638.097;1731.844;1825.568;1919.273]  Table=[400;500;600;700;800;900;1000;1100;1200;1300;1400;1500;1600;1700;1800;1900;2000]  InternalRulePriority=Speed  RndMeth=Simplest
  Out1 : Outport
  wires:
  In1/1 -> LUT 1.56RR/1
  LUT 1.56RR/1 -> Out1/1

== system LUT_liver_pancreas_30/If Action Subsystem6/If Action Subsystem2/If Action Subsystem6/If Action Subsystem6 ==
  In1 : Inport
  Action Port : ActionPort  ActionPortLabel=elseif( u1 >= 1.545)
  LUT 1.55RR : Lookup_n-D  NumberOfTableDimensions=1  BreakpointsForDimension1=[458.5649;506.6679;601.8856;697.074;791.9177;886.4833;980.8447;1075.056;1169.156;1263.172;1357.123;1451.022;1544.881;1638.708;1732.507;1826.284;1920.042]  Table=[400;500;600;700;800;900;1000;1100;1200;1300;1400;1500;1600;1700;1800;1900;2000]  InternalRulePriority=Speed  RndMeth=Simplest
  Out1 : Outport
  wires:
  In1/1 -> LUT 1.55RR/1
  LUT 1.55RR/1 -> Out1/1

== system LUT_liver_pancreas_30/If Action Subsystem6/If Action Subsystem2/If Action Subsystem6/If Action Subsystem7 ==
  In1 : Inport
  Action Port : ActionPort  ActionPortLabel=elseif( u1 >= 1.565)
  LUT 1.57RR : Lookup_n-D  NumberOfTableDimensions=1  BreakpointsForDimension1=[458.3885;506.505;601.6751;696.8004;791.5699;886.0534;980.3268;1074.446;1168.451;1262.368;1356.219;1450.018;1543.774;1637.497;1731.192;1824.865;1918.517]  Table=[400;500;600;700;800;900;1000;1100;1200;1300;1400;1500;1600;1700;1800;1900;2000]  InternalRulePriority=Speed  RndMeth=Simplest
  Out1 : Outport
  wires:
  In1/1 -> LUT 1.57RR/1
  LUT 1.57RR/1 -> Out1/1

== system LUT_liver_pancreas_30/If Action Subsystem6/If Action Subsystem2/If Action Subsystem6/If Action Subsystem8 ==
  In1 : Inport
  Action Port : ActionPort  ActionPortLabel=elseif(u1 >= 1.575)
  LUT 1.58RR : Lookup_n-D  NumberOfTableDimensions=1  BreakpointsForDimension1=[458.3021;506.4257;601.5729;696.6678;791.4014;885.8451;980.0756;1074.15;1168.108;1261.978;1355.78;1449.529;1543.235;1636.908;1730.552;1824.173;1917.774]  Table=[400;500;600;700;800;900;1000;1100;1200;1300;1400;1500;1600;1700;1800;1900;2000]  InternalRulePriority=Speed  RndMeth=Simplest
  Out1 : Outport
  wires:
  In1/1 -> LUT 1.58RR/1
  LUT 1.58RR/1 -> Out1/1

== system LUT_liver_pancreas_30/If Action Subsystem6/If Action Subsystem2/If Action Subsystem6/If Action Subsystem9 ==
  In1 : Inport
  Action Port : ActionPort  ActionPortLabel=if(u1 >= 1.585)
  LUT 1.59RR : Lookup_n-D  NumberOfTableDimensions=1  BreakpointsForDimension1=[458.2169;506.3477;601.4728;696.538;791.2364;885.6409;979.8294;1073.86;1167.772;1261.595;1355.349;1449.049;1542.706;1636.328;1729.922;1823.492;1917.043]  Table=[400;500;600;700;800;900;1000;1100;1200;1300;1400;1500;1600;1700;1800;1900;2000]  InternalRulePriority=Speed  RndMeth=Simplest
  Out1 : Outport
  wires:
  In1/1 -> LUT 1.59RR/1
  LUT 1.59RR/1 -> Out1/1

== system LUT_liver_pancreas_30/If Action Subsystem6/If Action Subsystem2/If Action Subsystem7/If Action Subsystem1 ==
  In1 : Inport
  Action Port : ActionPort  ActionPortLabel=elseif( u1 >= 1.715)
  LUT 1.72RR : Lookup_n-D  NumberOfTableDimensions=1  BreakpointsForDimension1=[457.2074;505.4439;600.3368;695.0767;789.3798;883.3376;977.0412;1070.558;1163.936;1257.207;1350.398;1443.524;1536.599;1629.632;1722.632;1815.605;1908.553]  Table=[400;500;600;700;800;900;1000;1100;1200;1300;1400;1500;1600;1700;1800;1900;2000]  InternalRulePriority=Speed  RndMeth=Simplest
  Out1 : Outport
  wires:
  In1/1 -> LUT 1.72RR/1
  LUT 1.72RR/1 -> Out1/1

== system LUT_liver_pancreas_30/If Action Subsystem6/If Action Subsystem2/If Action Subsystem7/If Action Subsystem10 ==
  In1 : Inport
  Action Port : ActionPort  ActionPortLabel=elseif( u1>= 1.705)
  LUT 1.71RR : Lookup_n-D  NumberOfTableDimensions=1  BreakpointsForDimension1=[457.2791;505.5068;600.4143;695.1755;789.5053;883.4936;977.2308;1070.783;1164.198;1257.509;1350.739;1443.905;1537.021;1630.097;1723.139;1816.153;1909.145]  Table=[400;500;600;700;800;900;1000;1100;1200;1300;1400;1500;1600;1700;1800;1900;2000]  InternalRulePriority=Speed  RndMeth=Simplest
  Out1 : Outport
  wires:
  In1/1 -> LUT 1.71RR/1
  LUT 1.71RR/1 -> Out1/1

== system LUT_liver_pancreas_30/If Action Subsystem6/If Action Subsystem2/If Action Subsystem7/If Action Subsystem2 ==
  In1 : Inport
  Action Port : ActionPort  ActionPortLabel=else
  LUT 1.70RR : Lookup_n-D  NumberOfTableDimensions=1  BreakpointsForDimension1=[457.3518;505.5707;600.4932;695.2764;789.6334;883.6529;977.4242;1071.013;1164.466;1257.816;1351.086;1444.293;1537.451;1630.569;1723.654;1816.711;1909.746]  Table=[400;500;600;700;800;900;1000;1100;1200;1300;1400;1500;1600;1700;1800;1900;2000]  InternalRulePriority=Speed  RndMeth=Simplest
  Out1 : Outport
  wires:
  In1/1 -> LUT 1.70RR/1
  LUT 1.70RR/1 -> Out1/1

== system LUT_liver_pancreas_30/If Action Subsystem6/If Action Subsystem2/If Action Subsystem7/If Action Subsystem3 ==
  In1 : Inport
  Action Port : ActionPort  ActionPortLabel=elseif( u1 >= 1.725)
  LUT 1.73RR : Lookup_n-D  NumberOfTableDimensions=1  BreakpointsForDimension1=[457.1366;505.382;600.2609;694.9799;789.257;883.1847;976.8554;1070.337;1163.678;1256.911;1350.063;1443.149;1536.183;1629.176;1722.134;1815.065;1907.971]  Table=[400;500;600;700;800;900;1000;1100;1200;1300;1400;1500;1600;1700;1800;1900;2000]  InternalRulePriority=Speed  RndMeth=Simplest
  Out1 : Outport
  wires:
  In1/1 -> LUT 1.73RR/1
  LUT 1.73RR/1 -> Out1/1

== system LUT_liver_pancreas_30/If Action Subsystem6/If Action Subsystem2/If Action Subsystem7/If Action Subsystem4 ==
  In1 : Inport
  Action Port : ActionPort  ActionPortLabel=elseif( u1 >= 1.735)
  LUT 1.74RR : Lookup_n-D  NumberOfTableDimensions=1  BreakpointsForDimension1=[457.0667;505.3211;600.1864;694.8851;789.1367;883.035;976.6733;1070.12;1163.425;1256.621;1349.733;1442.78;1535.775;1628.727;1721.645;1814.534;1907.399]  Table=[400;500;600;700;800;900;1000;1100;1200;1300;1400;1500;1600;1700;1800;1900;2000]  InternalRulePriority=Speed  RndMeth=Simplest
  Out1 : Outport
  wires:
  In1/1 -> LUT 1.74RR/1
  LUT 1.74RR/1 -> Out1/1

== system LUT_liver_pancreas_30/If Action Subsystem6/If Action Subsystem2/If Action Subsystem7/If Action Subsystem5 ==
  In1 : Inport
  Action Port : ActionPort  ActionPortLabel=elseif( u1 >= 1.755)
  LUT 1.76RR : Lookup_n-D  NumberOfTableDimensions=1  BreakpointsForDimension1=[456.9295;505.2022;600.0418;694.7015;788.9037;882.7448;976.32;1069.7;1162.933;1256.056;1349.093;1442.062;1534.978;1627.851;1720.689;1813.497;1906.28]  Table=[400;500;600;700;800;900;1000;1100;1200;1300;1400;1500;1600;1700;1800;1900;2000]  InternalRulePriority=Speed  RndMeth=Simplest
  Out1 : Outport
  wires:
  In1/1 -> LUT 1.76RR/1
  LUT 1.76RR/1 -> Out1/1

== system LUT_liver_pancreas_30/If Action Subsystem6/If Action Subsystem2/If Action Subsystem7/If Action Subsystem6 ==
  In1 : Inport
  Action Port : ActionPort  ActionPortLabel=elseif( u1 >= 1.745)
  LUT 1.75RR : Lookup_n-D  NumberOfTableDimensions=1  BreakpointsForDimension1=[456.9977;505.2612;600.1134;694.7923;789.019;882.8884;976.4949;1069.908;1163.177;1256.336;1349.41;1442.418;1535.373;1628.285;1721.163;1814.011;1906.835]  Table=[400;500;600;700;800;900;1000;1100;1200;1300;1400;1500;1600;1700;1800;1900;2000]  InternalRulePriority=Speed  RndMeth=Simplest
  Out1 : Outport
  wires:
  In1/1 -> LUT 1.75RR/1
  LUT 1.75RR/1 -> Out1/1

== system LUT_liver_pancreas_30/If Action Subsystem6/If Action Subsystem2/If Action Subsystem7/If Action Subsystem7 ==
  In1 : Inport
  Action Port : ActionPort  ActionPortLabel=elseif( u1 >= 1.765)
  LUT 1.77RR : Lookup_n-D  NumberOfTableDimensions=1  BreakpointsForDimension1=[456.8622;505.1441;599.9715;694.6125;788.7909;882.6042;976.1487;1069.495;1162.694;1255.781;1348.781;1441.713;1534.59;1627.424;1720.222;1812.99;1905.734]  Table=[400;500;600;700;800;900;1000;1100;1200;1300;1400;1500;1600;1700;1800;1900;2000]  InternalRulePriority=Speed  RndMeth=Simplest
  Out1 : Outport
  wires:
  In1/1 -> LUT 1.77RR/1
  LUT 1.77RR/1 -> Out1/1

== system LUT_liver_pancreas_30/If Action Subsystem6/If Action Subsystem2/If Action Subsystem7/If Action Subsystem8 ==
  In1 : Inport
  Action Port : ActionPort  ActionPortLabel=elseif(u1 >= 1.775)
  LUT 1.78RR : Lookup_n-D  NumberOfTableDimensions=1  BreakpointsForDimension1=[456.7957;505.0869;599.9026;694.5254;788.6804;882.4664;975.9807;1069.295;1162.46;1255.511;1348.475;1441.369;1534.209;1627.004;1719.763;1812.492;1905.196]  Table=[400;500;600;700;800;900;1000;1100;1200;1300;1400;1500;1600;1700;1800;1900;2000]  InternalRulePriority=Speed  RndMeth=Simplest
  Out1 : Outport
  wires:
  In1/1 -> LUT 1.78RR/1
  LUT 1.78RR/1 -> Out1/1

== system LUT_liver_pancreas_30/If Action Subsystem6/If Action Subsystem2/If Action Subsystem7/If Action Subsystem9 ==
  In1 : Inport
  Action Port : ActionPort  ActionPortLabel=if(u1 >= 1.785)
  LUT 1.79RR : Lookup_n-D  NumberOfTableDimensions=1  BreakpointsForDimension1=[456.73;505.0307;599.8351;694.4401;788.5722;882.3315;975.8162;1069.099;1162.23;1255.246;1348.174;1441.032;1533.834;1626.591;1719.312;1812.002;1904.667]  Table=[400;500;600;700;800;900;1000;1100;1200;1300;1400;1500;1600;1700;1800;1900;2000]  InternalRulePriority=Speed  RndMeth=Simplest
  Out1 : Outport
  wires:
  In1/1 -> LUT 1.79RR/1
  LUT 1.79RR/1 -> Out1/1

== system LUT_liver_pancreas_30/If Action Subsystem6/If Action Subsystem2/If Action Subsystem8/If Action Subsystem1 ==
  In1 : Inport
  Action Port : ActionPort  ActionPortLabel=elseif( u1 >= 1.815)
  LUT 1.82RR : Lookup_n-D  NumberOfTableDimensions=1  BreakpointsForDimension1=[456.5376;504.8669;599.64;694.1947;788.2613;881.9435;975.3421;1068.532;1161.565;1254.48;1347.303;1440.053;1532.746;1625.393;1718.001;1810.578;1903.129]  Table=[400;500;600;700;800;900;1000;1100;1200;1300;1400;1500;1600;1700;1800;1900;2000]  InternalRulePriority=Speed  RndMeth=Simplest
  Out1 : Outport
  wires:
  In1/1 -> LUT 1.82RR/1
  LUT 1.82RR/1 -> Out1/1

== system LUT_liver_pancreas_30/If Action Subsystem6/If Action Subsystem2/If Action Subsystem8/If Action Subsystem10 ==
  In1 : Inport
  Action Port : ActionPort  ActionPortLabel=elseif( u1>= 1.805)
  LUT 1.81RR : Lookup_n-D  NumberOfTableDimensions=1  BreakpointsForDimension1=[456.6009;504.9207;599.7038;694.2748;788.3628;882.0701;975.4969;1068.717;1161.782;1254.731;1347.588;1440.374;1533.103;1625.786;1718.431;1811.045;1903.634]  Table=[400;500;600;700;800;900;1000;1100;1200;1300;1400;1500;1600;1700;1800;1900;2000]  InternalRulePriority=Speed  RndMeth=Simplest
  Out1 : Outport
  wires:
  In1/1 -> LUT 1.81RR/1
  LUT 1.81RR/1 -> Out1/1

== system LUT_liver_pancreas_30/If Action Subsystem6/If Action Subsystem2/If Action Subsystem8/If Action Subsystem2 ==
  In1 : Inport
  Action Port : ActionPort  ActionPortLabel=else
  LUT 1.80RR : Lookup_n-D  NumberOfTableDimensions=1  BreakpointsForDimension1=[456.665;504.9752;599.7688;694.3566;788.4664;882.1995;975.6549;1068.906;1162.004;1254.986;1347.878;1440.7;1533.465;1626.185;1718.868;1811.52;1904.146]  Table=[400;500;600;700;800;900;1000;1100;1200;1300;1400;1500;1600;1700;1800;1900;2000]  InternalRulePriority=Speed  RndMeth=Simplest
  Out1 : Outport
  wires:
  In1/1 -> LUT 1.80RR/1
  LUT 1.80RR/1 -> Out1/1

== system LUT_liver_pancreas_30/If Action Subsystem6/If Action Subsystem2/If Action Subsystem8/If Action Subsystem3 ==
  In1 : Inport
  Action Port : ActionPort  ActionPortLabel=elseif( u1 >= 1.825)
  LUT 1.83RR : Lookup_n-D  NumberOfTableDimensions=1  BreakpointsForDimension1=[456.475;504.814;599.5775;694.1163;788.1621;881.8195;975.1904;1068.35;1161.352;1254.234;1347.022;1439.738;1532.396;1625.006;1717.578;1810.119;1902.632]  Table=[400;500;600;700;800;900;1000;1100;1200;1300;1400;1500;1600;1700;1800;1900;2000]  InternalRulePriority=Speed  RndMeth=Simplest
  Out1 : Outport
  wires:
  In1/1 -> LUT 1.83RR/1
  LUT 1.83RR/1 -> Out1/1

== system LUT_liver_pancreas_30/If Action Subsystem6/If Action Subsystem2/If Action Subsystem8/If Action Subsystem4 ==
  In1 : Inport
  Action Port : ActionPort  ActionPortLabel=elseif( u1 >= 1.835)
  LUT 1.84RR : Lookup_n-D  NumberOfTableDimensions=1  BreakpointsForDimension1=[456.4131;504.7619;599.5161;694.0396;788.0649;881.698;975.0418;1068.172;1161.143;1253.992;1346.747;1439.429;1532.051;1624.626;1717.162;1809.666;1902.143]  Table=[400;500;600;700;800;900;1000;1100;1200;1300;1400;1500;1600;1700;1800;1900;2000]  InternalRulePriority=Speed  RndMeth=Simplest
  Out1 : Outport
  wires:
  In1/1 -> LUT 1.84RR/1
  LUT 1.84RR/1 -> Out1/1

== system LUT_liver_pancreas_30/If Action Subsystem6/If Action Subsystem2/If Action Subsystem8/If Action Subsystem5 ==
  In1 : Inport
  Action Port : ActionPort  ActionPortLabel=elseif( u1 >= 1.855)
  LUT 1.86RR : Lookup_n-D  NumberOfTableDimensions=1  BreakpointsForDimension1=[456.2916;504.66;599.3969;693.8908;787.8768;881.4628;974.7536;1067.826;1160.736;1253.522;1346.211;1438.825;1531.379;1623.885;1716.35;1808.783;1901.188]  Table=[400;500;600;700;800;900;1000;1100;1200;1300;1400;1500;1600;1700;1800;1900;2000]  InternalRulePriority=Speed  RndMeth=Simplest
  Out1 : Outport
  wires:
  In1/1 -> LUT 1.86RR/1
  LUT 1.86RR/1 -> Out1/1

== system LUT_liver_pancreas_30/If Action Subsystem6/If Action Subsystem2/If Action Subsystem8/If Action Subsystem6 ==
  In1 : Inport
  Action Port : ActionPort  ActionPortLabel=elseif( u1 >= 1.845)
  LUT 1.85RR : Lookup_n-D  NumberOfTableDimensions=1  BreakpointsForDimension1=[456.352;504.7106;599.4559;693.9644;787.9699;881.5792;974.8962;1067.998;1160.937;1253.755;1346.477;1439.124;1531.712;1624.252;1716.753;1809.221;1901.662]  Table=[400;500;600;700;800;900;1000;1100;1200;1300;1400;1500;1600;1700;1800;1900;2000]  InternalRulePriority=Speed  RndMeth=Simplest
  Out1 : Outport
  wires:
  In1/1 -> LUT 1.85RR/1
  LUT 1.85RR/1 -> Out1/1

== system LUT_liver_pancreas_30/If Action Subsystem6/If Action Subsystem2/If Action Subsystem8/If Action Subsystem7 ==
  In1 : Inport
  Action Port : ActionPort  ActionPortLabel=elseif( u1 >= 1.865)
  LUT 1.87RR : Lookup_n-D  NumberOfTableDimensions=1  BreakpointsForDimension1=[456.2319;504.6102;599.339;693.8188;787.7858;881.3489;974.6138;1067.659;1160.539;1253.293;1345.951;1438.532;1531.052;1623.523;1715.954;1808.351;1900.721]  Table=[400;500;600;700;800;900;1000;1100;1200;1300;1400;1500;1600;1700;1800;1900;2000]  InternalRulePriority=Speed  RndMeth=Simplest
  Out1 : Outport
  wires:
  In1/1 -> LUT 1.87RR/1
  LUT 1.87RR/1 -> Out1/1

== system LUT_liver_pancreas_30/If Action Subsystem6/If Action Subsystem2/If Action Subsystem8/If Action Subsystem8 ==
  In1 : Inport
  Action Port : ActionPort  ActionPortLabel=elseif(u1 >= 1.875)
  LUT 1.88RR : Lookup_n-D  NumberOfTableDimensions=1  BreakpointsForDimension1=[456.1729;504.5612;599.2822;693.7483;787.6967;881.2374;974.477;1067.494;1160.345;1253.069;1345.694;1438.243;1530.73;1623.167;1715.564;1807.927;1900.261]  Table=[400;500;600;700;800;900;1000;1100;1200;1300;1400;1500;1600;1700;1800;1900;2000]  InternalRulePriority=Speed  RndMeth=Simplest
  Out1 : Outport
  wires:
  In1/1 -> LUT 1.88RR/1
  LUT 1.88RR/1 -> Out1/1

== system LUT_liver_pancreas_30/If Action Subsystem6/If Action Subsystem2/If Action Subsystem8/If Action Subsystem9 ==
  In1 : Inport
  Action Port : ActionPort  ActionPortLabel=if(u1 >= 1.885)
  LUT 1.89RR : Lookup_n-D  NumberOfTableDimensions=1  BreakpointsForDimension1=[456.1145;504.5128;599.2265;693.6793;787.6095;881.1282;974.3429;1067.333;1160.155;1252.848;1345.443;1437.959;1530.413;1622.817;1715.18;1807.509;1899.809]  Table=[400;500;600;700;800;900;1000;1100;1200;1300;1400;1500;1600;1700;1800;1900;2000]  InternalRulePriority=Speed  RndMeth=Simplest
  Out1 : Outport
  wires:
  In1/1 -> LUT 1.89RR/1
  LUT 1.89RR/1 -> Out1/1
